simulink model "SECTION10_2"  (R2018b)
settings: Solver=FixedStepDiscrete  StartTime=0.0  StopTime=10.0  RelTol=1e-3
undefined symbols (not defined in the file or in its folder): DiscIntNeverNeededParam
libraries: simulink x1
settings Model: DataTypeOverride=Off  MinMaxOverflowArchiveMode=Merge  Creator=ESPINO NOTEBOOK  LastModifiedBy=ESPINO NOTEBOOK
settings DataIOCC: LimitDataPoints=on  SaveOutput=off  SaveTime=off
settings OptimizationCC: BlockReduction=off  ConditionallyExecuteInputs=off  DefaultParameterBehavior=Inlined  LifeSpan=inf
settings DebuggingCC: AlgebraicLoopMsg=error  SingleTaskRateTransMsg=error  AllowSymbolicDim=off  StrictBusMsg=ErrorOnBusTreatedAsVector  SFUnexpectedBacktrackingDiag=warning  SFNoUnconditionalDefaultTransitionDiag=warning  SFExecutionAtInitializationDiag=none
settings HardwareCC: ProdBitPerPointer=32  ProdBitPerSizeT=32  ProdBitPerPtrDiffT=32  ProdLargestAtomicFloat=None  ProdIntDivRoundTo=Undefined  ProdEndianess=Unspecified  ProdWordSize=32  ProdHWDeviceType=ASIC/FPGA->ASIC/FPGA  ProdEqTarget=off
settings SFSimCC: SimUseLocalCustomCode=off
settings RTWCC: RTWUseLocalCustomCode=off
settings CodeAppCC: StateflowObjectComments=on
settings GRTTargetCC: TargetLangStandard=C89/C90 (ANSI)  GeneratePreprocessorConditionals=Disable all
settings ConfigComp: CovScope=ReferencedModels  CovMetricSettings=dw  CovHtmlReporting=on  CovSaveCumulativeToWorkspaceVar=on  CovSaveSingleToWorkspaceVar=on  CovExternalEMLEnable=off  CovSFcnEnable=off

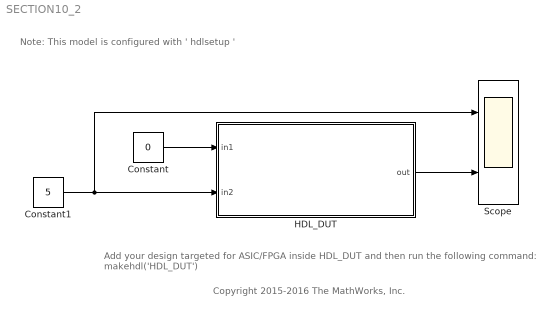
== system SECTION10_2 ==
  note: Note: This model is configured with ' hdlsetup '
  note: Add your design targeted for ASIC/FPGA inside HDL_DUT and then run the following command:
      | makehdl('HDL_DUT')
  note: Copyright 2015-2016 The MathWorks, Inc.
  Constant : Constant  Value=0  OutDataTypeStr=fixdt(0,4,0)  SampleTime=0.01
  Constant1 : Constant  Value=5  OutDataTypeStr=fixdt(1,32,10)  SampleTime=0.01
  HDL_DUT : Subsystem
  Scope : Scope  NumInputPorts=2
  wires:
  Constant/1 -> HDL_DUT/1(in1)
  Constant1/1 -> Scope/1, HDL_DUT/2(in2)
  HDL_DUT/1(out) -> Scope/2

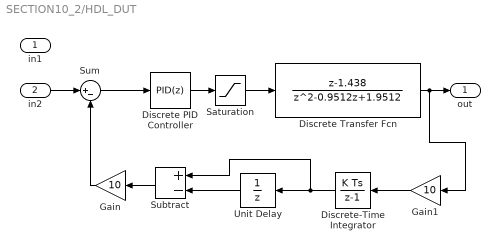
== system SECTION10_2/HDL_DUT ==
  in1 : Inport
  in2 : Inport  Port=2  OutDataTypeStr=fixdt(1,32,10)  SampleTime=0.01
  Discrete Transfer Fcn : DiscreteTransferFcn  Numerator="[1  -1.438]"  Denominator="[1  -0.9512   1.9512]"  SampleTime=0.01  StateDataTypeStr=fixdt(1,32,10)  NumCoefDataTypeStr=fixdt(1,32,10)  DenCoefDataTypeStr=fixdt(1,32,10)  NumProductDataTypeStr=fixdt(1,32,10)  DenProductDataTypeStr=fixdt(1,32,10)  NumAccumDataTypeStr=fixdt(1,32,10)  DenAccumDataTypeStr=fixdt(1,32,10)  OutDataTypeStr=fixdt(1,32,10)
  Discrete PID Controller : simulink/Continuous/PID Controller  Controller=PID  Form=Parallel  TimeDomain=Discrete-time  SampleTime=0.01  IntegratorMethod=Forward Euler  FilterMethod=Forward Euler  ControllerParametersSource=internal  P=0.10  I=0.6426  D=0.00047  UseFilter=on  N=20.74  TunerSelectOption=Transfer Function Based (PID Tuner App)  InitialConditionSource=internal  InitialConditionForIntegrator=0  InitialConditionForFilter=0  DifferentiatorICPrevScaledInput=0  ExternalReset=none  TrackingMode=off  Kt=1  LimitOutput=off  UpperSaturationLimit=inf  LowerSaturationLimit=-inf  LinearizeAsGain=off  AntiWindupMode=none  Kb=1  RndMeth=Round  PGainOutDataTypeStr=fixdt(1,32,10)  PProdOutDataTypeStr=fixdt(1,32,10)  POutMin=[]  POutMax=[]  IGainOutDataTypeStr=fixdt(1,32,10)  IProdOutDataTypeStr=fixdt(1,32,10)  IOutMin=[]  IOutMax=[]  DGainOutDataTypeStr=fixdt(1,32,10)  DProdOutDataTypeStr=fixdt(1,32,10)  DOutMin=[]  DOutMax=[]  NGainOutDataTypeStr=fixdt(1,32,10)  NProdOutDataTypeStr=fixdt(1,32,10)  NOutMin=[]  NOutMax=[]  SumOutDataTypeStr=fixdt(1,32,10)  SumOutMin=[]  SumOutMax=[]  SaturationOutMin=[]  SaturationOutMax=[]  PParamDataTypeStr=fixdt(1,32,10)  PParamMin=[]  PParamMax=[]  IParamDataTypeStr=fixdt(1,32,10)  IParamMin=[]  IParamMax=[]  DParamDataTypeStr=fixdt(1,32,10)  DParamMin=[]  DParamMax=[]  NParamDataTypeStr=fixdt(1,32,10)  NParamMin=[]  NParamMax=[]  KbParamMin=[]  KbParamMax=[]  KtParamMin=[]  KtParamMax=[]  KbOutMin=[]  KbOutMax=[]  KtOutMin=[]  KtOutMax=[]  IntegratorOutDataTypeStr=fixdt(1,32,10)  IntegratorOutMin=[]  IntegratorOutMax=[]  FilterOutDataTypeStr=fixdt(1,32,10)  FilterOutMin=[]  FilterOutMax=[]  SumI1OutMin=[]  SumI1OutMax=[]  SumI2OutMin=[]  SumI2OutMax=[]  SumI3OutMin=[]  SumI3OutMax=[]  SumI4OutMin=[]  SumI4OutMax=[]  SumDOutDataTypeStr=fixdt(1,32,10)  SumDOutMin=[]  SumDOutMax=[]  SumAccumDataTypeStr=fixdt(1,32,10)  SumDAccumDataTypeStr=fixdt(1,32,10)  DifferentiatorOutMin=[]  DifferentiatorOutMax=[]  FilterDiffOutCoefMin=[]  FilterDiffOutCoefMax=[]  ReciprocalOutMin=[]  ReciprocalOutMax=[]  SumDenOutMin=[]  SumDenOutMax=[]  SumNumOutMin=[]  SumNumOutMax=[]  DivideOutMin=[]  DivideOutMax=[]  IntegratorContinuousStateAttributes=''  IntegratorStateMustResolveToSignalObject=off  IntegratorRTWStateStorageClass=Auto  FilterContinuousStateAttributes=''  FilterStateMustResolveToSignalObject=off  FilterRTWStateStorageClass=Auto  ParallelPVariant=InternalParameters  IdealPVariant=Disabled  IVariant=InternalParameters  DVariant=InternalParameters  IntegratorVariant=Discrete  SatVariant=Disabled  AWVariant=Passthrough  PCopyVariant=Disabled  TRVariant=Disabled  FdbkBlocksVariant=Forward  IdealPFdbkVariant=Disabled  SatFdbkVariant=Disabled  DerivativeFilterVariant=ForwardEulerFilter  NVariant=InternalParameters  NCopyVariant=Disabled  FilterICVariant=InternalICsFilter  IntegratorICVariant=InternalICs  ExternalResetVariant=Disabled  TRSumVariant=Passthrough  SumFdbkVariant=Disabled  SumVariant=Sum_PID
  Discrete-Time Integrator : DiscreteIntegrator  gainval=1  SampleTime=0.01  OutDataTypeStr=fixdt(1,32,10)  ICPrevOutput=DiscIntNeverNeededParam  ICPrevScaledInput=DiscIntNeverNeededParam
  Gain : Gain  Gain=10  OutDataTypeStr=fixdt(1,32,10)
  Gain1 : Gain  Gain=10  OutDataTypeStr=fixdt(1,32,10)
  Saturation : Saturate  UpperLimit=100  LowerLimit=0  OutDataTypeStr=fixdt(1,32,10)
  Subtract : Sum  Inputs=+-  OutDataTypeStr=fixdt(1,32,10)
  Sum : Sum  Inputs=|+-  AccumDataTypeStr=fixdt(1,32,10)  OutDataTypeStr=fixdt(1,32,10)
  Unit Delay : UnitDelay  SampleTime=0.01
  out : Outport
  wires:
  Discrete-Time Integrator/1 -> Subtract/1, Unit Delay/1
  Unit Delay/1 -> Subtract/2
  Gain1/1 -> Discrete-Time Integrator/1
  Subtract/1 -> Gain/1
  Gain/1 -> Sum/2
  Discrete PID Controller/1 -> Saturation/1
  Sum/1 -> Discrete PID Controller/1
  in2/1 -> Sum/1
  Discrete Transfer Fcn/1 -> Gain1/1, out/1
  Saturation/1 -> Discrete Transfer Fcn/1
